simulink model "Encoder_reader_simulink"  (R2025a)
settings: Solver=FixedStepAuto  StartTime=0.0  StopTime=inf  FixedStep=0.001  RelTol=1e-3  EnableMultiTasking=on
libraries: stm32g4xxblockslib x1
settings Model: STM32="{\"EncoderBlockForG4\":[{\"ID\":\"untitled:1\"},{\"ID\":\"Lab3_Encoder:1\"}]}"  Creator=User  LastModifiedBy=ItsMoa
settings OptimizationCC: DefaultParameterBehavior=Inlined  EnhancedBackFolding=on  PassReuseOutputArgsAs=Individual arguments  ZeroExternalMemoryAtStartup=off  ZeroInternalMemoryAtStartup=off  MaxStackSize=512  OptimizeBlockOrder=speed  DifferentSizesBufferReuse=on  OptimizationCustomize=off  EfficientTunableParamExpr=on
settings DebuggingCC: ParameterTunabilityLossMsg=error
settings HardwareCC: ProdBitPerPointer=32.0  ProdBitPerSizeT=32.0  ProdBitPerPtrDiffT=32.0  ProdLargestAtomicInteger=Long  ProdLargestAtomicFloat=Double  ProdWordSize=32.0  ProdLongLongMode=on  ProdHWDeviceType=ARM Compatible->ARM Cortex-M
settings SFSimCC: MATLABDynamicMemAlloc=off
settings RTWCC: SystemTargetFile=ert.tlc  HardwareBoard=STM32G4xx Based  TemplateMakefile=ert_default_tmf  Toolchain=GNU Tools for ARM Embedded Processors  Description=Embedded Coder
settings CodeAppCC: ForceParamTrailComments=on  IgnoreCustomStorageClasses=off  OperatorAnnotations=on  SimulinkDataObjDesc=on  SFDataObjDesc=on  InsertBlockDesc=on
settings ERTTargetCC: ExtModeTransport=3.0  ExtModeStaticAllocSize=2048.0  TargetLangStandard=C99 (ISO)  CodeReplacementLibrary=ARM Cortex-M  SupportContinuousTime=on

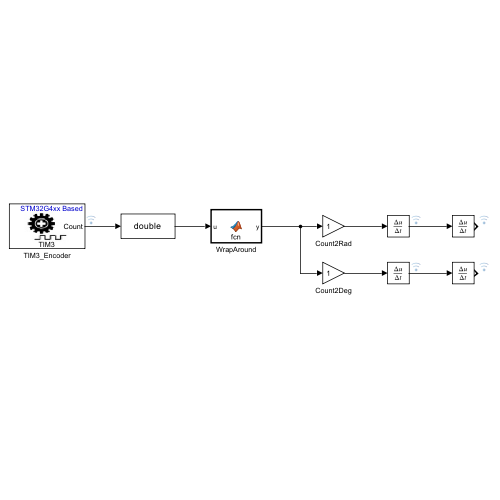
[thumbnail: Simulink's stored preview of the top-level diagram]
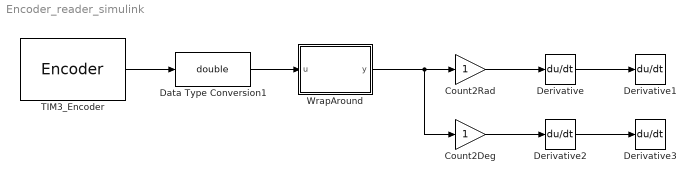
== system Encoder_reader_simulink ==
  Count2Deg : Gain
  Count2Rad : Gain
  Data Type Conversion1 : DataTypeConversion  OutDataTypeStr=double  SaturateOnIntegerOverflow=off  RndMeth=Floor
  Derivative{,1..3} (4 alike) : Derivative
  TIM3_Encoder : stm32g4xxblockslib/Encoder  TimerModule=TIM3  EnableResetInput=off  OutputCountAfterFirstIndex=off  OutputValidIndex=off  OutputDirection=off  OutputStatus=off  SampleTime=-1
  WrapAround : MATLAB Function  TreatAsAtomicUnit=on
  wires:
  TIM3_Encoder/1 -> Data Type Conversion1/1
  Data Type Conversion1/1 -> WrapAround/1(u)
  Derivative/1 -> Derivative1/1
  WrapAround/1(y) -> Count2Rad/1, Count2Deg/1
  Count2Rad/1 -> Derivative/1
  Count2Deg/1 -> Derivative2/1
  Derivative2/1 -> Derivative3/1

== matlab function Encoder_reader_simulink/WrapAround ==
  data: u input; y output
function y = fcn(u)

y = u;
